simulink model "ParamEstimatebb"  (R2016b)
settings: Solver=VariableStepAuto  StartTime=0.0  StopTime=time  RelTol=1e-3
settings Model: Creator=rrooijmans  LastModifiedBy=rrooijmans

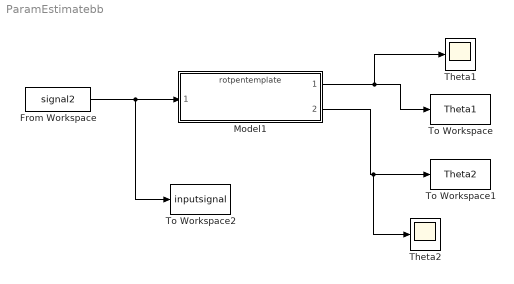
== system ParamEstimatebb ==
  From Workspace : FromWorkspace  VariableName=signal2  SampleTime=0
  Model1 : ModelReference  ModelNameDialog=rotpentemplate.slx  SimulationMode=Normal  ModelReferenceVersion=1.426
  Theta1 : Scope
  Theta2 : Scope
  To Workspace : ToWorkspace  VariableName=Theta1  SaveFormat=Timeseries  SampleTime=-1
  To Workspace1 : ToWorkspace  VariableName=Theta2  SaveFormat=Timeseries  SampleTime=-1
  To Workspace2 : ToWorkspace  VariableName=inputsignal  SaveFormat=Timeseries  SampleTime=-1
  wires:
  Model1/1 -> Theta1/1, To Workspace/1
  Model1/2 -> Theta2/1, To Workspace1/1
  From Workspace/1 -> To Workspace2/1, Model1/1
